simulink model "ALOHA_CSMA_Model"  (R2021b)
settings: Solver=FixedStepDiscrete  StartTime=0  StopTime=1  FixedStep=1  RelTol=1e-3
settings Model: Creator=Artem  LastModifiedBy=Dmitry

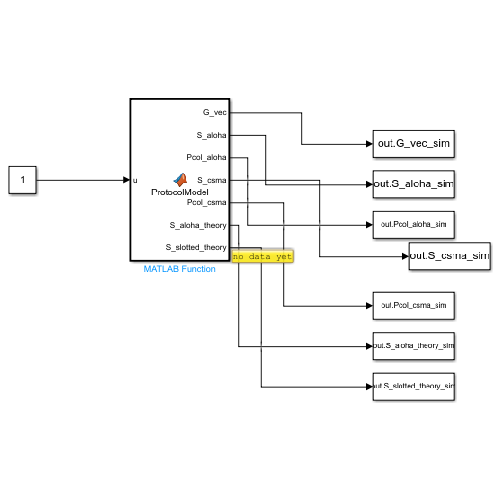
[thumbnail: Simulink's stored preview of the top-level diagram]
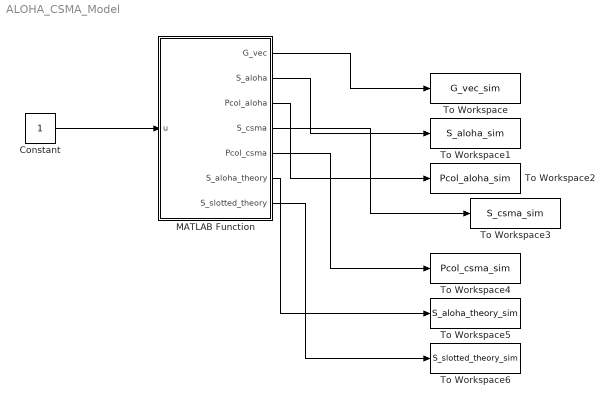
== system ALOHA_CSMA_Model ==
  Constant : Constant
  MATLAB Function : MATLAB Function  TreatAsAtomicUnit=on
  To Workspace : ToWorkspace  VariableName=G_vec_sim  SampleTime=-1
  To Workspace1 : ToWorkspace  VariableName=S_aloha_sim  SampleTime=-1
  To Workspace2 : ToWorkspace  VariableName=Pcol_aloha_sim  SampleTime=-1
  To Workspace3 : ToWorkspace  VariableName=S_csma_sim  SampleTime=-1
  To Workspace4 : ToWorkspace  VariableName=Pcol_csma_sim  SampleTime=-1
  To Workspace5 : ToWorkspace  VariableName=S_aloha_theory_sim  SampleTime=-1
  To Workspace6 : ToWorkspace  VariableName=S_slotted_theory_sim  SampleTime=-1
  wires:
  Constant/1 -> MATLAB Function/1(u)
  MATLAB Function/1(G_vec) -> To Workspace/1
  MATLAB Function/2(S_aloha) -> To Workspace1/1
  MATLAB Function/3(Pcol_aloha) -> To Workspace2/1
  MATLAB Function/4(S_csma) -> To Workspace3/1
  MATLAB Function/5(Pcol_csma) -> To Workspace4/1
  MATLAB Function/6(S_aloha_theory) -> To Workspace5/1
  MATLAB Function/7(S_slotted_theory) -> To Workspace6/1

== matlab function ALOHA_CSMA_Model/MATLAB Function ==
  data: u input; G_vec output; S_aloha output; Pcol_aloha output; S_csma output; Pcol_csma output; S_aloha_theory output; S_slotted_theory output
function [G_vec, S_aloha, Pcol_aloha, S_csma, Pcol_csma, S_aloha_theory, S_slotted_theory] = ProtocolModel(u)
%#codegen

T_packet = 1;
T_sim = 3000;
tau = 0.01 * T_packet;
backoffMax = 1 * T_packet;

nPoints = 20;

G_vec = zeros(1, 20);
S_aloha = zeros(1, 20);
Pcol_aloha = zeros(1, 20);
S_csma = zeros(1, 20);
Pcol_csma = zeros(1, 20);
S_aloha_theory = zeros(1, 20);
S_slotted_theory = zeros(1, 20);

for i = 1:nPoints
    G_vec(i) = 0.1 + (i - 1) * (4 - 0.1) / (nPoints - 1);
end

for i = 1:nPoints
    G = G_vec(i);

    [S_aloha(i), Pcol_aloha(i)] = pureAlohaSimple(G, T_sim, T_packet);
    [S_csma(i), Pcol_csma(i)] = csmaSimple(G, T_sim, T_packet, tau, backoffMax);

    S_aloha_theory(i) = G * exp(-2 * G);
    S_slotted_theory(i) = G * exp(-G);
end

end


function [S, P_collision] = pureAlohaSimple(G, T_sim, T_packet)

maxPackets = 20000;
arrivalTimes = zeros(maxPackets, 1);

currentTime = 0;
count = 0;

while currentTime < T_sim && count < maxPackets
    interArrivalTime = -log(rand()) / G;
    currentTime = currentTime + interArrivalTime;

    if currentTime < T_sim
        count = count + 1;
        arrivalTimes(count) = currentTime;
    end
end

if count == 0
    S = 0;
    P_collision = 0;
    return;
end

collided = false(maxPackets, 1);

for k = 1:count
    if k > 1
        if arrivalTimes(k) - arrivalTimes(k - 1) < T_packet
            collided(k) = true;
        end
    end

    if k < count
        if arrivalTimes(k + 1) - arrivalTimes(k) < T_packet
            collided(k) = true;
        end
    end
end

successfulPackets = 0;
collidedPackets = 0;

for k = 1:count
    if collided(k)
        collidedPackets = collidedPackets + 1;
    else
        successfulPackets = successfulPackets + 1;
    end
end

S = successfulPackets * T_packet / T_sim;
P_collision = collidedPackets / count;

end


function [S, P_collision] = csmaSimple(G, T_sim, T_packet, tau, backoffMax)

maxEvents = 50000;
eventTimes = zeros(maxEvents, 1);

currentTime = 0;
eventCount = 0;

while currentTime < T_sim && eventCount < maxEvents
    interArrivalTime = -log(rand()) / G;
    currentTime = currentTime + interArrivalTime;

    if currentTime < T_sim
        eventCount = eventCount + 1;
        eventTimes(eventCount) = currentTime;
    end
end

successfulPackets = 0;
collidedPackets = 0;
totalStartedTransmissions = 0;
channelBusyUntil = 0;

while eventCount > 0
    minTime = eventTimes(1);
    minIndex = 1;

    for i = 2:eventCount
        if eventTimes(i) < minTime
            minTime = eventTimes(i);
            minIndex = i;
        end
    end

    t = minTime;

    eventTimes(minIndex) = eventTimes(eventCount);
    eventTimes(eventCount) = 0;
    eventCount = eventCount - 1;

    if t > T_sim
        break;
    end

    if t < channelBusyUntil
        newAttemptTime = channelBusyUntil + rand() * backoffMax;

        if newAttemptTime <= T_sim && eventCount < maxEvents
            eventCount = eventCount + 1;
            eventTimes(eventCount) = newAttemptTime;
        end

        continue;
    end

    numberOfTransmitters = 1;
    latestStart = t;

    i = 1;
    while i <= eventCount
        if eventTimes(i) <= t + tau
            numberOfTransmitters = numberOfTransmitters + 1;

            if eventTimes(i) > latestStart
                latestStart = eventTimes(i);
            end
            

            eventTimes(i) = eventTimes(eventCount);
            eventTimes(eventCount) = 0;
            eventCount = eventCount - 1;
        else
            i = i + 1;
        end
    end

    totalStartedTransmissions = totalStartedTransmissions + numberOfTransmitters;
    channelBusyUntil = latestStart + T_packet;

    if numberOfTransmitters == 1
        successfulPackets = successfulPackets + 1;
    else
        collidedPackets = collidedPackets + numberOfTransmitters;
    end
end

S = successfulPackets * T_packet / T_sim;

if totalStartedTransmissions == 0
    P_collision = 0;
else
    P_collision = collidedPackets / totalStartedTransmissions;
end

end
